simulink model "tester"  (R2025b)
settings: Solver=ode4  StartTime=0.0  StopTime=Ttotal  FixedStep=0.001  RelTol=1e-3
values from neighbouring files (symbols this model uses):
  Ka = 1/20    (= 0.05)    [runGasSim.m]    (also in runGasSim2.m)
  Ki_Pm = Kp_Pm / a    (= 0)    [runGasSim.m]    (also in runGasSim2.m)
  Ki_Q2 = Kp_Q2 / a    (= 0)    [runGasSim.m]    (also in runGasSim2.m)
  Kp_Pm = Kp_vec_Pm(k)    [runGasSim.m]    (also in runGasSim2.m)
  Kp_Q2 = Kp_vec_Q2(k)    [runGasSim.m]    (also in runGasSim2.m)
  Ks1 = 20/(60-0)    (= 0.333333333333)    [runGasSim.m]    (also in runGasSim2.m)
  Ks2 = 20/(60-0)    (= 0.333333333333)    [runGasSim.m]    (also in runGasSim2.m)
  mode = 1    [runGasSim.m]    (also in runGasSim2.m)
  Pm_max = P1    (= 40)    [runGasSim.m]    (also in runGasSim2.m)
  Pm_min = 0    [runGasSim.m]    (also in runGasSim2.m)
  Pm_ref = 20    [runGasSim.m]    (also in runGasSim2.m)
  Q1 = Qout - Q2_ref    (= 8.33333333333)    [runGasSim.m]    (also in runGasSim2.m)
  Q2_ref = 1*1000/60    (= 16.6666666667)    [runGasSim.m]    (also in runGasSim2.m)
  s1int = funCV(cv1,false)    [runGasSim.m]    (also in runGasSim2.m)
  s2int = funCV(cv2,false)    [runGasSim.m]    (also in runGasSim2.m)
  SG = 0.6    [runGasSim.m]    (also in runGasSim2.m)
  T = 0.5    [runGasSim.m]    (also in runGasSim2.m)
  u_max = 1    [runGasSim.m]    (also in runGasSim2.m)
  u_min = 0    [runGasSim.m]    (also in runGasSim2.m)
settings Model: Creator=hannahgingery  LastModifiedBy=hannahgingery

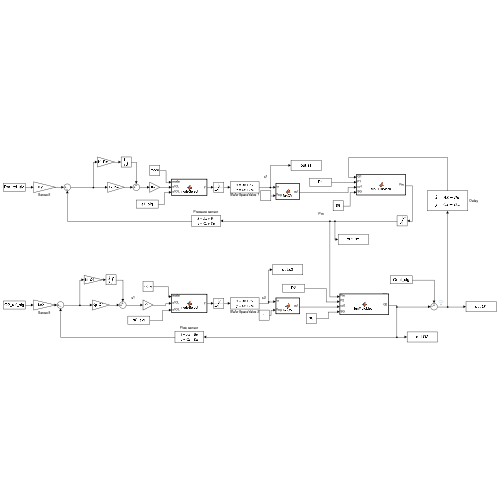
[thumbnail: Simulink's stored preview of the top-level diagram]
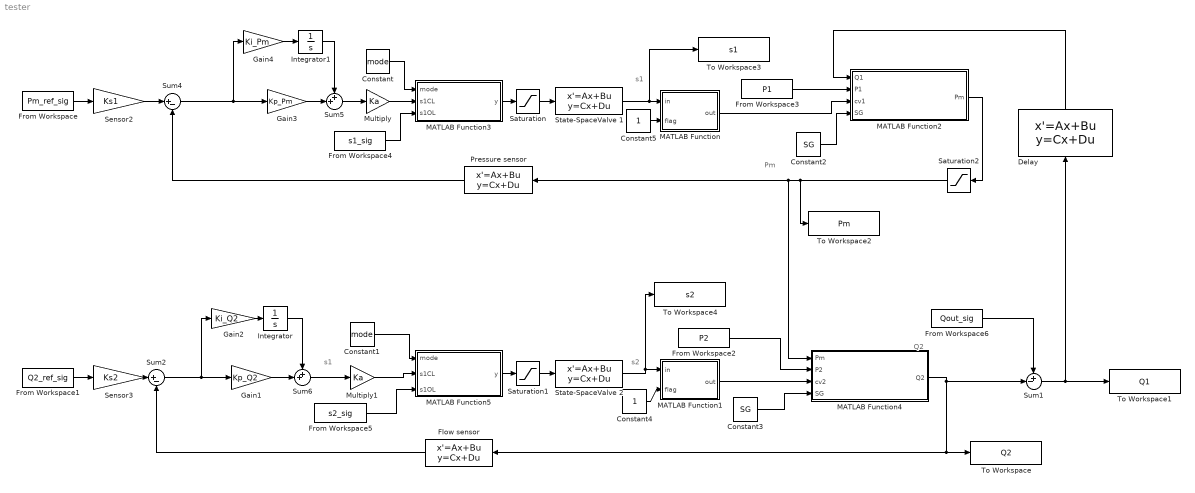
== system tester ==
  note: Pm
  note: s2
  note: s1
  note: s1
  note: Q2
  Constant : Constant  Value=mode
  Constant1 : Constant  Value=mode
  Constant2 : Constant  Value=SG
  Constant3 : Constant  Value=SG
  Constant4 : Constant
  Constant5 : Constant
  Delay : StateSpace  A=-20/T  B=20/T  D=0  InitialCondition=Q1
  Flow sensor : StateSpace  A=-10/T  B=Ks2*10/T  D=0  InitialCondition=Ks2*Q2_ref
  From Workspace : FromWorkspace  VariableName=Pm_ref_sig
  From Workspace1 : FromWorkspace  VariableName=Q2_ref_sig
  From Workspace2 : FromWorkspace  VariableName=P2
  From Workspace3 : FromWorkspace  VariableName=P1
  From Workspace4 : FromWorkspace  VariableName=s1_sig
  From Workspace5 : FromWorkspace  VariableName=s2_sig
  From Workspace6 : FromWorkspace  VariableName=Qout_sig
  Gain1 : Gain  Gain=Kp_Q2
  Gain2 : Gain  Gain=Ki_Q2
  Gain3 : Gain  Gain=Kp_Pm
  Gain4 : Gain  Gain=Ki_Pm
  Integrator : Integrator  InitialCondition=s2int/Ka  LimitOutput=on  UpperSaturationLimit=u_max/Ka  LowerSaturationLimit=u_min
  Integrator1 : Integrator  InitialCondition=s1int/Ka  LimitOutput=on  UpperSaturationLimit=u_max/Ka  LowerSaturationLimit=u_min
  MATLAB Function : MATLAB Function  TreatAsAtomicUnit=on
  MATLAB Function1 : MATLAB Function  TreatAsAtomicUnit=on
  MATLAB Function2 : MATLAB Function  TreatAsAtomicUnit=on
  MATLAB Function3 : MATLAB Function  TreatAsAtomicUnit=on
  MATLAB Function4 : MATLAB Function  TreatAsAtomicUnit=on
  MATLAB Function5 : MATLAB Function  TreatAsAtomicUnit=on
  Multiply : Gain  Gain=Ka
  Multiply1 : Gain  Gain=Ka
  Pressure sensor : StateSpace  A=-10/T  B=Ks1*10/T  D=0  InitialCondition=Pm_ref*Ks1
  Saturation : Saturate  UpperLimit=u_max  LowerLimit=u_min
  Saturation1 : Saturate  UpperLimit=u_max  LowerLimit=u_min
  Saturation2 : Saturate  UpperLimit=Pm_max  LowerLimit=Pm_min
  Sensor2 : Gain  Gain=Ks1
  Sensor3 : Gain  Gain=Ks2
  State-SpaceValve 1 : StateSpace  A=-1/T  B=1/T  D=0  InitialCondition=s1int
  State-SpaceValve 2 : StateSpace  A=-1/T  B=1/T  D=0  InitialCondition=s2int
  Sum1 : Sum  Inputs=+-|
  Sum2 : Sum  Inputs=|+-
  Sum4 : Sum  Inputs=|+-
  Sum5 : Sum  Inputs=++|
  Sum6 : Sum  Inputs=++|
  To Workspace : ToWorkspace  VariableName=Q2  SampleTime=-1
      settings: Save2DSignal=2-D array (concatenate along first dimension)
  To Workspace1 : ToWorkspace  VariableName=Q1  SampleTime=-1
      settings: Save2DSignal=2-D array (concatenate along first dimension)
  To Workspace2 : ToWorkspace  VariableName=Pm  SampleTime=-1
      settings: Save2DSignal=2-D array (concatenate along first dimension)
  To Workspace3 : ToWorkspace  VariableName=s1  SampleTime=-1
      settings: Save2DSignal=2-D array (concatenate along first dimension)
  To Workspace4 : ToWorkspace  VariableName=s2  SampleTime=-1
      settings: Save2DSignal=2-D array (concatenate along first dimension)
  wires:
  MATLAB Function4/1(Q2) -> Flow sensor/1, To Workspace/1, Sum1/2
  Sum6/1 -> Multiply1/1
  From Workspace4/1 -> MATLAB Function3/3(s1OL)
  Gain4/1 -> Integrator1/1
  Sum2/1 -> Gain2/1, Gain1/1
  From Workspace1/1 -> Sensor3/1
  Sensor2/1 -> Sum4/1
  Saturation1/1 -> State-SpaceValve 2/1
  Gain3/1 -> Sum5/2
  State-SpaceValve 2/1 -> To Workspace4/1, MATLAB Function1/1(in)
  From Workspace2/1 -> MATLAB Function4/2(P2)
  Constant4/1 -> MATLAB Function1/2(flag)
  MATLAB Function2/1(Pm) -> Saturation2/1
  Sum1/1 -> To Workspace1/1, Delay/1
  MATLAB Function5/1(y) -> Saturation1/1
  Sum4/1 -> Gain4/1, Gain3/1
  Gain2/1 -> Integrator/1
  Multiply1/1 -> MATLAB Function5/2(s1CL)
  MATLAB Function3/1(y) -> Saturation/1
  Integrator/1 -> Sum6/1
  Flow sensor/1 -> Sum2/2
  From Workspace5/1 -> MATLAB Function5/3(s1OL)
  Gain1/1 -> Sum6/2
  Saturation/1 -> State-SpaceValve 1/1
  Integrator1/1 -> Sum5/1
  From Workspace6/1 -> Sum1/1
  From Workspace/1 -> Sensor2/1
  Pressure sensor/1 -> Sum4/2
  Constant5/1 -> MATLAB Function/2(flag)
  Sensor3/1 -> Sum2/1
  Constant3/1 -> MATLAB Function4/4(SG)
  Multiply/1 -> MATLAB Function3/2(s1CL)
  Constant/1 -> MATLAB Function3/1(mode)
  State-SpaceValve 1/1 -> To Workspace3/1, MATLAB Function/1(in)
  Saturation2/1 -> Pressure sensor/1, MATLAB Function4/1(Pm), To Workspace2/1
  Constant1/1 -> MATLAB Function5/1(mode)
  From Workspace3/1 -> MATLAB Function2/2(P1)
  Delay/1 -> MATLAB Function2/1(Q1)
  MATLAB Function/1(out) -> MATLAB Function2/3(cv1)
  Constant2/1 -> MATLAB Function2/4(SG)
  MATLAB Function1/1(out) -> MATLAB Function4/3(cv2)
  Sum5/1 -> Multiply/1

== matlab function tester/MATLAB Function1 ==
  data: in input; out output; flag input
function out  = funCV(in,flag)
%If flag is true,
%   in = stem position (0 to 1)
%   out = Cv
%else
%   in = Cv
%   out = stem position

sd = [0:0.1:1]';
cvd = [0; 0.84; 1.49; 6.68; 12.3; 17.3; 22.1; 26.7; 30.9; 34.4; 36.1];

if flag %stem is input, cv is output
    if any(in<(-eps) | in>(1+eps)); error('stem position must be between 0 and 1'); end
    out = interp1(sd,cvd,in,'linear');
else
    if any(in>(max(cvd)+eps) | in<-eps); error('Cv range error'); end
    out = interp1(cvd,sd,in,'linear');
end

%Cv = (5e-7) .* u.^4 - 0.0002.*u.^3 + 0.0179.*u.^2 - 0.1729.*u +0.1748;

%0.0000005.*u*exp(4)-0.0002.*u*exp(3)+0.0179.*u.*exp(2)-0.1729.*u+0.1748;
end

== matlab function tester/MATLAB Function ==
  data: in input; out output; flag input
function out  = funCV(in,flag)
%If flag is true,
%   in = stem position (0 to 1)
%   out = Cv
%else
%   in = Cv
%   out = stem position

sd = [0:0.1:1]';
cvd = [0; 0.84; 1.49; 6.68; 12.3; 17.3; 22.1; 26.7; 30.9; 34.4; 36.1];

if flag %stem is input, cv is output
    if any(in<(-eps) | in>(1+eps)); error('stem position must be between 0 and 1'); end
    out = interp1(sd,cvd,in,'linear');
else
    if any(in>(max(cvd)+eps) | in<-eps); error('Cv range error'); end
    out = interp1(cvd,sd,in,'linear');
end

%Cv = (5e-7) .* u.^4 - 0.0002.*u.^3 + 0.0179.*u.^2 - 0.1729.*u +0.1748;

%0.0000005.*u*exp(4)-0.0002.*u*exp(3)+0.0179.*u.*exp(2)-0.1729.*u+0.1748;
end

== matlab function tester/MATLAB Function2 ==
  data: Q1 input; P1 input; Pm output; cv1 input; SG input
function Pm  = funFluidMech(Q1,P1,cv1,SG)

Pm = P1- (Q1/cv1)^2 *SG;

end

== matlab function tester/MATLAB Function3 ==
  data: mode input; y output; s1CL input; s1OL input
function y = modeSelect(mode, s1CL, s1OL)
% mode: 1 = CL, 0 = OL

    if mode == 1
        y = s1CL;
    else
        y = s1OL;
    end
end

== matlab function tester/MATLAB Function4 ==
  data: Pm input; P2 input; Q2 output; cv2 input; SG input
function Q2  = funFluidMech(Pm,P2,cv2,SG)

Q2 = cv2*sqrt((P2-Pm)/SG);

end

== matlab function tester/MATLAB Function5 ==
  data: mode input; y output; s1CL input; s1OL input
function y = modeSelect(mode, s1CL, s1OL)
% mode: 1 = CL, 0 = OL

    if mode == 1
        y = s1CL;
    else
        y = s1OL;
    end
end
